simulink model "DEP_PROJECT"  (R2022b)
settings: Solver=VariableStepAuto  StartTime=0.0  StopTime=2
undefined symbols (not defined in the file): Ion, Lithium
libraries: spsMosfetLib x6, spsBatteryLib x1, spsPermanentMagnetSynchronousMachineLib x1, simulink x1, slpidlib x1, spspowerguiLib x1
settings Model: Creator=Deepak  LastModifiedBy=revat
settings SolverCC: AlgebraicLoopSolver=TrustRegion
settings DebuggingCC: UnconnectedInputMsg=warning  UnconnectedOutputMsg=warning  UnconnectedLineMsg=warning  SFMachineParentedDataDiag=warning
settings ModelReferenceCC: EnableRefExpFcnMdlSchedulingChecks=on
settings SFSimCC: CustomCodeUndefinedFunction=UseInterfaceOnly

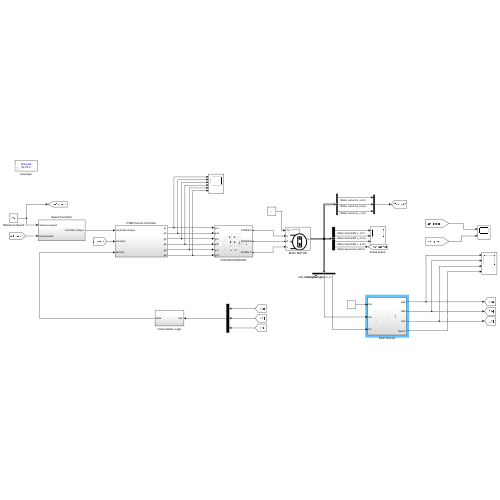
[thumbnail: Simulink's stored preview of the top-level diagram]
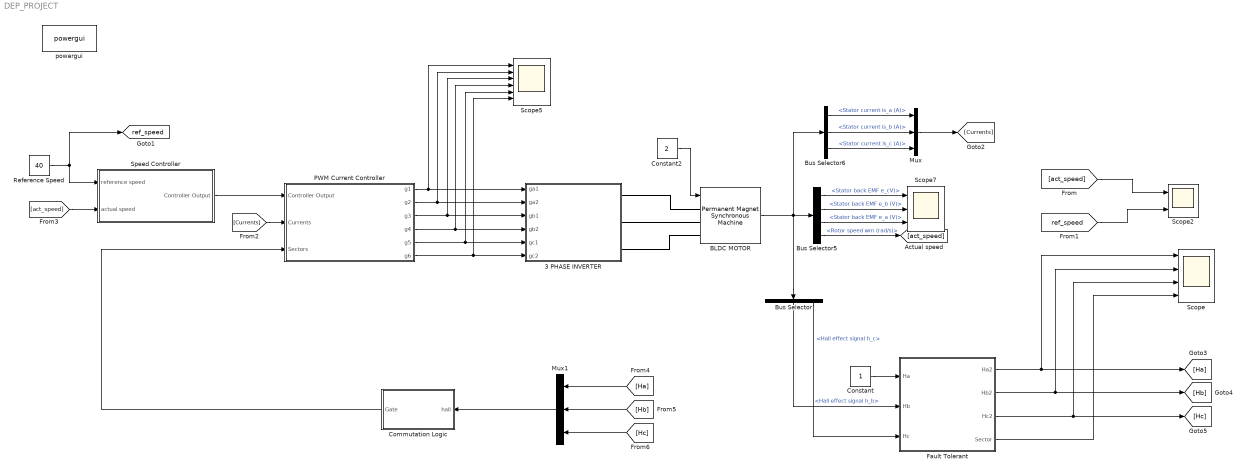
== system DEP_PROJECT ==
  3 PHASE INVERTER : Subsystem
  BLDC MOTOR : spsPermanentMagnetSynchronousMachineLib/Permanent Magnet Synchronous Machine  NbPhases=3  FluxDistribution=Trapezoidal  RotorType=Round  MechanicalLoad=Torque Tm  PresetModel=No  ShowDetailedParameters=on  MeasurementBus=off  Resistance=0.7  Inductance=2.7e-3  dqInductances=[8.5e-3,8.5e-3]  La=0.000395  MachineConstant=Flux linkage established by magnets (V.s)  Flux=0.1194  VoltageCst=100.0283  TorqueCst=0.9552  Flat=120  Mechanical=[0.0027 0.0004924 4 0]  PolePairs=4  InitialConditions=[0,0, 0,0]  InitialConditions5ph=[0 0 0 0 0 0]  RefAngle=90 degrees behind phase A axis (modified Park)  IterativeDiscreteModel=Trapezoidal non iterative  TsBlock=-1  TsPowergui=0
  Bus Selector : BusSelector  OutputSignals=Hall effect signal h_a,Hall effect signal h_b,Hall effect signal h_c
  Bus Selector5 : BusSelector  OutputSignals=Stator back EMF e_cV),Stator back EMF e_b (V),Stator back EMF e_a (V),Rotor speed wm (rad/s)
  Bus Selector6 : BusSelector  OutputSignals=Stator current is_a (A),Stator current is_b (A),Stator current is_c (A)
  Commutation Logic : Subsystem
  Constant : Constant
  Constant2 : Constant  Value=2
  Fault Tolerant : Subsystem
  Mux : Mux  Inputs=3
  Mux1 : Mux  Inputs=3
  PWM Current Controller : Subsystem
  Reference Speed : Constant  Value=40
  Scope : Scope  NumInputPorts=4
  Scope2 : Scope  NumInputPorts=2
  Scope5 : Scope  NumInputPorts=6
  Scope7 : Scope  NumInputPorts=3
  Speed Controller : Subsystem
  powergui : spspowerguiLib/powergui  Priority=1  SimulationMode=Discrete  SampleTime=50e-6  frequency=60  Iterations=50  frequencyindice=0  Pbase=100e6  ErrMax=1e-4  UnitsV=kV  UnitsW=MW  buscounter=0  FunctionMessages=off  echomessages=off  EnableUseOfTLC=off  CurrentSourceSwitches=off  DisableSnubberDevices=off  DisableRonSwitches=off  DisableVfSwitches=off  DisplayEquations=off  AutomaticDiscreteSolvers=off  SolverType=Tustin/Backward Euler (TBE)  Interpol=off  ExternalGateDelay=off  methode=off  Ts=100  x0status=blocks  SPID=on  SwTol=0  HookPort=off  NonlinearTolerance=0  nMaxIteration=15  ContinueOnMaxIteration=off  RestoreLinks=warning  ResistiveCurrentMeasurement=off  Frange=[0:2:500]  Ylog=off  Xlog=on  ShowGrid=off  save=off  variable=ZData  structure=0  ZoomFFT=off  StartTime=0.0  cycles=1  DisplayStyle=1  fundamental=60  FreqAxis=off  MaxFrequency=1000  frequencyindicesteady=1  RmsSteady=1  display=off
  tag scope: ref_speed=global
  wires:
  Constant2/1 -> BLDC MOTOR/1
  PWM Current Controller/3(g3) -> Scope5/3, 3 PHASE INVERTER/3(gb1)
  PWM Current Controller/2(g2) -> 3 PHASE INVERTER/2(ga2), Scope5/2
  Commutation Logic/1(Gate) -> PWM Current Controller/3(Sectors)
  Bus Selector6/3 -> Mux/3  "<Stator current is_c (A)>"
  Bus Selector6/2 -> Mux/2  "<Stator current is_b (A)>"
  Reference Speed/1 -> Speed Controller/1(reference speed), [ref_speed]
  Speed Controller/1("Controller Output ") -> PWM Current Controller/1("Controller Output ")
  Bus Selector5/3 -> Scope7/3  "<Stator back EMF e_a (V)>"
  PWM Current Controller/5(g5) -> Scope5/5, 3 PHASE INVERTER/5(gc1)
  Bus Selector5/2 -> Scope7/2  "<Stator back EMF e_b (V)>"
  Bus Selector6/1 -> Mux/1  "<Stator current is_a (A)>"
  PWM Current Controller/6(g6) -> 3 PHASE INVERTER/6(gc2), Scope5/6
  PWM Current Controller/4(g4) -> Scope5/4, 3 PHASE INVERTER/4(gb2)
  Bus Selector5/4 -> [act_speed]  "<Rotor speed wm (rad/s)>"
  BLDC MOTOR/1 -> Bus Selector5/1, Bus Selector/1, Bus Selector6/1
  PWM Current Controller/1(g1) -> 3 PHASE INVERTER/1(ga1), Scope5/1
  Bus Selector5/1 -> Scope7/1  "<Stator back EMF e_cV)>"
  Mux1/1 -> Commutation Logic/1("hall ")
  [act_speed] -> Scope2/1
  [Currents] -> PWM Current Controller/2(Currents)
  Mux/1 -> [Currents]
  [act_speed] -> Speed Controller/2(actual speed)
  Fault Tolerant/1(Ha2) -> Scope/1, [Ha]
  Fault Tolerant/2(Hb2) -> [Hb], Scope/2
  Fault Tolerant/3(Hc2) -> [Hc], Scope/3
  Fault Tolerant/4(Sector) -> Scope/4
  Bus Selector/3 -> Fault Tolerant/3(Hc)  "<Hall effect signal h_c>"
  [Ha] -> Mux1/1
  [Hb] -> Mux1/2
  [Hc] -> Mux1/3
  [ref_speed] -> Scope2/2
  Bus Selector/2 -> Fault Tolerant/2(Hb)  "<Hall effect signal h_b>"
  Constant/1 -> Fault Tolerant/1(Ha)
  connections:
  3 PHASE INVERTER/RConn3 -- BLDC MOTOR/LConn3
  3 PHASE INVERTER/RConn1 -- BLDC MOTOR/LConn1
  3 PHASE INVERTER/RConn2 -- BLDC MOTOR/LConn2

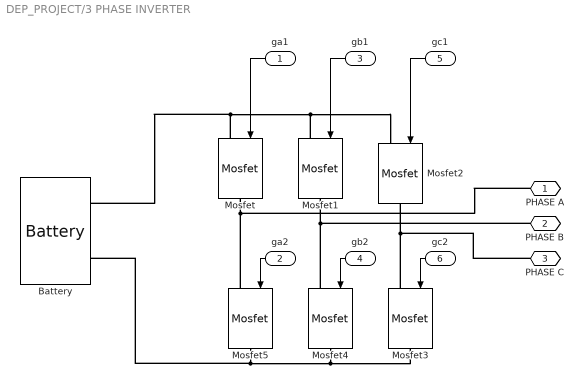
== system DEP_PROJECT/3 PHASE INVERTER ==
  ga1 : Inport
  ga2 : Inport  Port=2
  gb1 : Inport  Port=3
  gb2 : Inport  Port=4
  gc1 : Inport  Port=5
  gc2 : Inport  Port=6
  Battery : spsBatteryLib/Battery  BatType=Lithium-Ion  ShowTempParam=off  ThermalPreset=no  ShowAgeParam=off  NomV=48  NomQ=80  SOC=60  Batt_Tr=30  PresetModel=off  MaxQ=84  MinV=36  FullV=56.818272  Dis_rate=27.82608  R=0.006  Normal_OP=57.87524  expZone=[54.89208 3.144344]  current=[1.5 3]  Units=Ampere-hour  Tci=20  NomT=20  T2=-30  MaxQ2=4.8  FullV2=7.1  Normal_OP2=5.655  expZone2="[6.58           1]"  Rca=0.6  ti=2000  Dp=0  Neq0=0  Tsim=1e6  Ta1=25  Qeol=5.4*0.9  Reol=0.013333*1.2  Char_age=[2.3478, 3]  Dis_age=[2.3478, 10]  N1=1500  N2=10500  N3=1000  N4=1400  Ta2=45  N5=950
  Mosfet{,1..5} (6 alike) : spsMosfetLib/Mosfet  Ron=0.1  Lon=0  Rd=0.01  Vfd=0  IC=0  Rs=1e5  Cs=inf  Measurements=off
  PHASE A : PMIOPort  Side=Right
  PHASE B : PMIOPort  Port=2  Side=Right
  PHASE C : PMIOPort  Port=3  Side=Right
  wires:
  ga1/1 -> Mosfet/1
  ga2/1 -> Mosfet5/1
  gb1/1 -> Mosfet1/1
  gb2/1 -> Mosfet4/1
  gc1/1 -> Mosfet2/1
  gc2/1 -> Mosfet3/1
  connections:
  Mosfet5/LConn1 -- PHASE A/RConn1 -- Mosfet/RConn1
  PHASE B/RConn1 -- Mosfet4/LConn1 -- Mosfet1/RConn1
  Mosfet3/LConn1 -- PHASE C/RConn1 -- Mosfet2/RConn1
  Mosfet5/RConn1 -- Battery/LConn2 -- Mosfet4/RConn1 -- Mosfet3/RConn1
  Mosfet/LConn1 -- Battery/LConn1 -- Mosfet1/LConn1 -- Mosfet2/LConn1

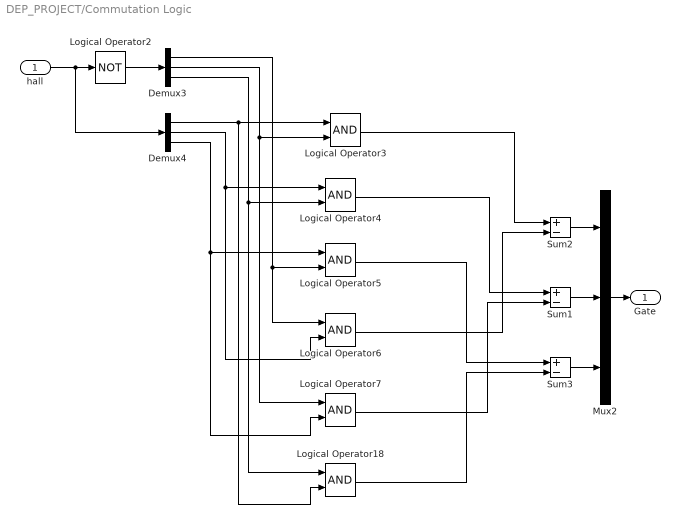
== system DEP_PROJECT/Commutation Logic ==
  "hall " : Inport
  Demux3 : Demux  Outputs=3
  Demux4 : Demux  Outputs=3
  Logical Operator{3..7,18} (6 alike) : Logic  AllPortsSameDT=off  OutDataTypeStr=boolean
  Logical Operator2 : Logic  Operator=NOT  AllPortsSameDT=off  OutDataTypeStr=boolean
  Mux2 : Mux  Inputs=3
  Sum1 : Sum  Inputs=+-  OutDataTypeStr=double
  Sum2 : Sum  Inputs=+-  OutDataTypeStr=double
  Sum3 : Sum  Inputs=+-  OutDataTypeStr=double
  Gate : Outport  VectorParamsAs1DForOutWhenUnconnected=off
  wires:
  Demux3/3 -> Logical Operator18/1, Logical Operator4/2
  Logical Operator6/1 -> Sum2/2
  Mux2/1 -> Gate/1
  Logical Operator7/1 -> Sum1/2
  Logical Operator4/1 -> Sum1/1
  Demux4/1 -> Logical Operator18/2, Logical Operator3/1
  Sum2/1 -> Mux2/1
  Demux4/3 -> Logical Operator5/1, Logical Operator7/2
  Demux4/2 -> Logical Operator4/1, Logical Operator6/2
  Logical Operator5/1 -> Sum3/1
  Logical Operator3/1 -> Sum2/1
  Sum1/1 -> Mux2/2
  Demux3/1 -> Logical Operator5/2, Logical Operator6/1
  Logical Operator2/1 -> Demux3/1
  Logical Operator18/1 -> Sum3/2
  Demux3/2 -> Logical Operator7/1, Logical Operator3/2
  "hall "/1 -> Logical Operator2/1, Demux4/1
  Sum3/1 -> Mux2/3

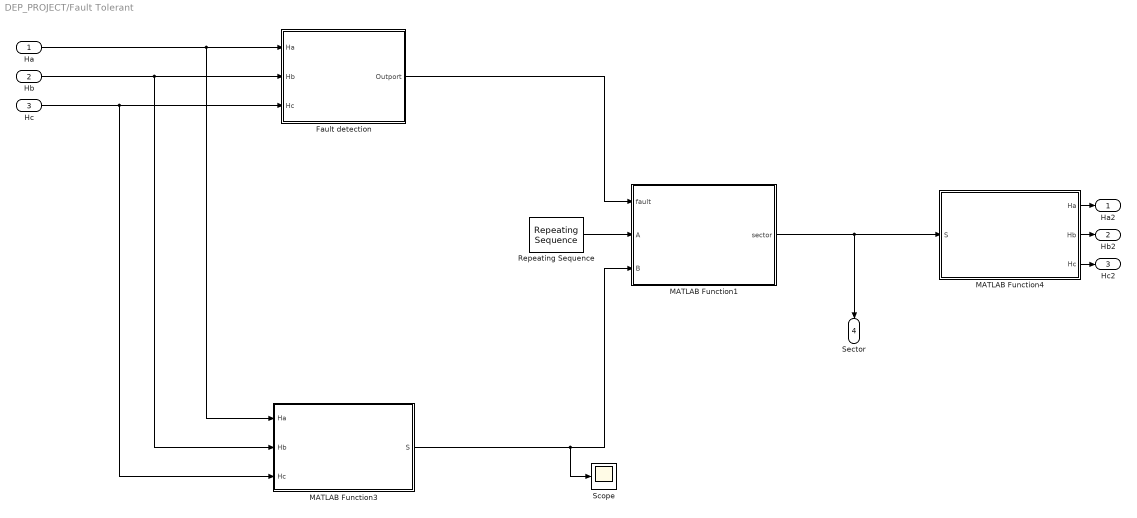
== system DEP_PROJECT/Fault Tolerant ==
  Ha : Inport
  Hb : Inport  Port=2
  Hc : Inport  Port=3
  Fault detection : Subsystem
  MATLAB Function1 : MATLAB Function  TreatAsAtomicUnit=on
  MATLAB Function3 : MATLAB Function  TreatAsAtomicUnit=on
  MATLAB Function4 : MATLAB Function  TreatAsAtomicUnit=on
  Repeating Sequence : simulink/Sources/Repeating Sequence  rep_seq_t=[0 8.799 8.8 17.59999 17.6 26.39999 26.4 35.1999 35.2 43.9999 44 52.79999 52.8]*(6.616/8.8)*1e-03  rep_seq_y=[1 1 2 2 3 3 4 4 5 5 6 6 1]
  Scope : Scope
  Ha2 : Outport
  Hb2 : Outport  Port=2
  Hc2 : Outport  Port=3
  Sector : Outport  Port=4
  wires:
  Hb/1 -> MATLAB Function3/2(Hb), Fault detection/2(Hb)
  Fault detection/1(Outport) -> MATLAB Function1/1(fault)
  MATLAB Function3/1(S) -> Scope/1, MATLAB Function1/3(B)
  MATLAB Function4/3(Hc) -> Hc2/1
  Hc/1 -> MATLAB Function3/3(Hc), Fault detection/3(Hc)
  MATLAB Function4/1(Ha) -> Ha2/1
  MATLAB Function1/1(sector) -> Sector/1, MATLAB Function4/1(S)
  Ha/1 -> MATLAB Function3/1(Ha), Fault detection/1(Ha)
  MATLAB Function4/2(Hb) -> Hb2/1
  Repeating Sequence/1 -> MATLAB Function1/2(A)

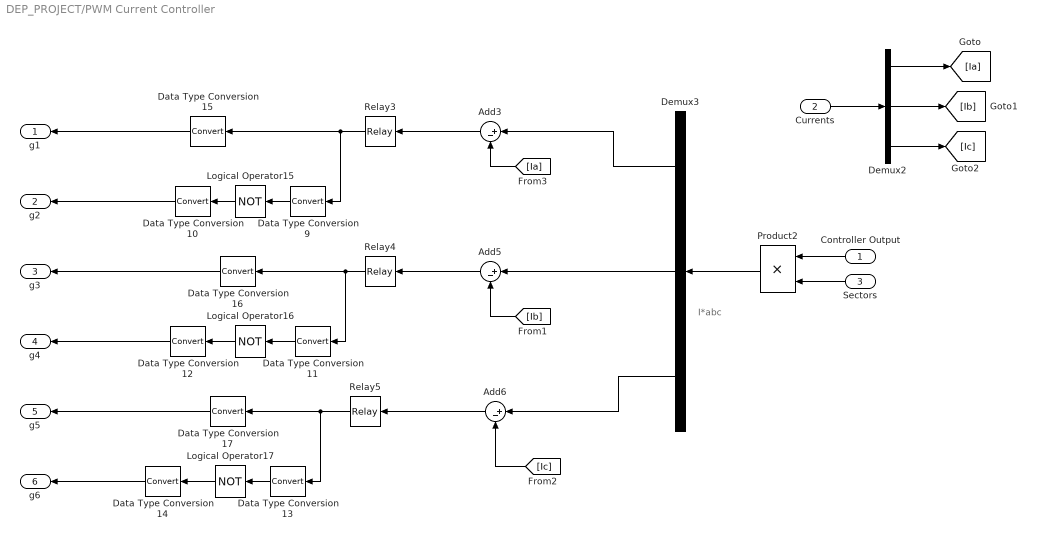
== system DEP_PROJECT/PWM Current Controller ==
  note: I*abc
  "Controller Output " : Inport
  Currents : Inport  Port=2
  Sectors : Inport  Port=3
  Add3 : Sum  Inputs=|+-
  Add5 : Sum  Inputs=|+-
  Add6 : Sum  Inputs=|+-
  Data Type Conversion{9..17} (9 alike) : DataTypeConversion
  Demux2 : Demux  Outputs=3
  Demux3 : Demux  Outputs=3
      settings: DisplayOption=none
  Logical Operator15 : Logic  Operator=NOT  AllPortsSameDT=off  OutDataTypeStr=boolean
  Logical Operator16 : Logic  Operator=NOT  AllPortsSameDT=off  OutDataTypeStr=boolean
  Logical Operator17 : Logic  Operator=NOT  AllPortsSameDT=off  OutDataTypeStr=boolean
  Product2 : Product  SaturateOnIntegerOverflow=on  OutDataTypeStr=Inherit: Same as first input
  Relay3 : Relay  OnSwitchValue=0.1  OffSwitchValue=-0.1
  Relay4 : Relay  OnSwitchValue=0.1  OffSwitchValue=-0.1
  Relay5 : Relay  OnSwitchValue=0.1  OffSwitchValue=-0.1
  g1 : Outport  VectorParamsAs1DForOutWhenUnconnected=off
  g2 : Outport  Port=2  VectorParamsAs1DForOutWhenUnconnected=off
  g3 : Outport  Port=3  VectorParamsAs1DForOutWhenUnconnected=off
  g4 : Outport  Port=4  VectorParamsAs1DForOutWhenUnconnected=off
  g5 : Outport  Port=5  VectorParamsAs1DForOutWhenUnconnected=off
  g6 : Outport  Port=6  VectorParamsAs1DForOutWhenUnconnected=off
  wires:
  Currents/1 -> Demux2/1
  Demux2/1 -> [Ia]
  Demux2/2 -> [Ib]
  Demux2/3 -> [Ic]
  "Controller Output "/1 -> Product2/1
  Sectors/1 -> Product2/2
  Add6/1 -> Relay5/1
  Add5/1 -> Relay4/1
  Demux3/1 -> Add3/1
  Data Type Conversion16/1 -> g3/1
  Data Type Conversion13/1 -> Logical Operator17/1
  Add3/1 -> Relay3/1
  Product2/1 -> Demux3/1
  Relay3/1 -> Data Type Conversion15/1, Data Type Conversion9/1
  Data Type Conversion15/1 -> g1/1
  Relay4/1 -> Data Type Conversion16/1, Data Type Conversion11/1
  Data Type Conversion17/1 -> g5/1
  Data Type Conversion12/1 -> g4/1
  Data Type Conversion10/1 -> g2/1
  Data Type Conversion11/1 -> Logical Operator16/1
  [Ic] -> Add6/2
  Logical Operator17/1 -> Data Type Conversion14/1
  Data Type Conversion14/1 -> g6/1
  Demux3/2 -> Add5/1
  Relay5/1 -> Data Type Conversion17/1, Data Type Conversion13/1
  Logical Operator15/1 -> Data Type Conversion10/1
  Logical Operator16/1 -> Data Type Conversion12/1
  [Ia] -> Add3/2
  Demux3/3 -> Add6/1
  Data Type Conversion9/1 -> Logical Operator15/1
  [Ib] -> Add5/2

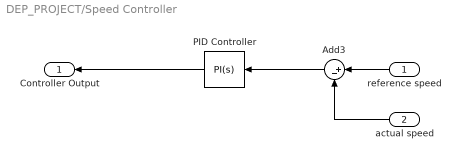
== system DEP_PROJECT/Speed Controller ==
  reference speed : Inport
  actual speed : Inport  Port=2
  Add3 : Sum  Inputs=|+-
  PID Controller : slpidlib/PID Controller  Controller=PI  Form=Parallel  TimeDomain=Continuous-time  UseExternalTs=off  SampleTime=-1  IntegratorMethod=Forward Euler  FilterMethod=Forward Euler  ControllerParametersSource=internal  P=5  I=4.9  UseKiTs=off  D=0  N=100  UseFilter=on  TunerSelectOption=Transfer Function Based (PID Tuner App)  InitialConditionSource=internal  InitialConditionForIntegrator=0  InitialConditionForFilter=0  DifferentiatorICPrevScaledInput=0  ExternalReset=none  TrackingMode=off  Kt=1  LimitOutput=off  SatLimitsSource=internal  UpperSaturationLimit=10  LowerSaturationLimit=0  LinearizeAsGain=on  AntiWindupMode=none  Kb=1  LimitIntegrator=off  UpperIntegratorSaturationLimit=inf  LowerIntegratorSaturationLimit=-inf  POutMin=[]  POutMax=[]  IOutMin=[]  IOutMax=[]  DOutMin=[]  DOutMax=[]  NOutMin=[]  NOutMax=[]  SumOutMin=[]  SumOutMax=[]  SaturationOutMin=[]  SaturationOutMax=[]  PParamMin=[]  PParamMax=[]  IParamMin=[]  IParamMax=[]  DParamMin=[]  DParamMax=[]  NParamMin=[]  NParamMax=[]  KbParamMin=[]  KbParamMax=[]  KtParamMin=[]  KtParamMax=[]  KbOutMin=[]  KbOutMax=[]  KtOutMin=[]  KtOutMax=[]  IntegratorOutMin=[]  IntegratorOutMax=[]  FilterOutMin=[]  FilterOutMax=[]  SumI1OutMin=[]  SumI1OutMax=[]  SumI2OutMin=[]  SumI2OutMax=[]  SumI3OutMin=[]  SumI3OutMax=[]  SumI4OutMin=[]  SumI4OutMax=[]  SumDOutMin=[]  SumDOutMax=[]  DifferentiatorOutMin=[]  DifferentiatorOutMax=[]  FilterDiffOutCoefMin=[]  FilterDiffOutCoefMax=[]  ReciprocalOutMin=[]  ReciprocalOutMax=[]  SumDenOutMin=[]  SumDenOutMax=[]  SumNumOutMin=[]  SumNumOutMax=[]  DivideOutMin=[]  DivideOutMax=[]  UdiffTsProdOutMin=[]  UdiffTsProdOutMax=[]  NTsProdOutMin=[]  NTsProdOutMax=[]  UintegralTsProdOutMin=[]  UintegralTsProdOutMax=[]  UngainTsProdOutMin=[]  UngainTsProdOutMax=[]  ClampingZeroOutDataTypeStr=Inherit: Inherit via back propagation  ClampingZeroOutMin=[]  ClampingZeroOutMax=[]  FilterDenConstantOutDataTypeStr=Inherit: Inherit via back propagation  FilterDenConstantOutMin=[]  FilterDenConstantOutMax=[]  PCopyOutDataTypeStr=Inherit: Inherit via back propagation  PCopyOutMin=[]  PCopyOutMax=[]  NCopyOutDataTypeStr=Inherit: Inherit via back propagation  NCopyOutMin=[]  NCopyOutMax=[]  IntegratorContinuousStateAttributes=''  IntegratorStateMustResolveToSignalObject=off  IntegratorRTWStateStorageClass=Auto  FilterContinuousStateAttributes=''  FilterStateMustResolveToSignalObject=off  FilterRTWStateStorageClass=Auto  ParallelPVariant=InternalParameters  IdealPVariant=Disabled  IVariant=InternalParameters  DVariant=Disabled  IntegratorVariant=Continuous  SatVariant=Disabled  AWVariant=Passthrough  PCopyVariant=Disabled  TRVariant=Disabled  FdbkBlocksVariant=Forward  IdealPFdbkVariant=Disabled  SatFdbkVariant=Disabled  DerivativeFilterVariant=Disabled  NVariant=Disabled  NCopyVariant=Disabled_SignalSpec  FilterICVariant=Disabled  IntegratorICVariant=InternalICs  ExternalResetVariant=Disabled  TRSumVariant=Passthrough  SumFdbkVariant=Disabled  SumVariant=Sum_PI  TsampFilterVariant=InternalTs  TsampNgainVariant=Passthrough  TsampIntegralVariant=Passthrough  ExternalSaturationOutDataTypeStr=Inherit: Same as second input
  "Controller Output " : Outport  VectorParamsAs1DForOutWhenUnconnected=off
  wires:
  Add3/1 -> PID Controller/1
  actual speed/1 -> Add3/2
  PID Controller/1 -> "Controller Output "/1
  reference speed/1 -> Add3/1

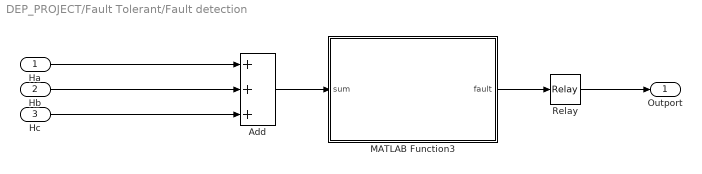
== system DEP_PROJECT/Fault Tolerant/Fault detection ==
  Ha : Inport
  Hb : Inport  Port=2
  Hc : Inport  Port=3
  Add : Sum  Inputs=+++
  MATLAB Function3 : MATLAB Function  TreatAsAtomicUnit=on
  Relay : Relay  OnSwitchValue=1  OffSwitchValue=-1
  Outport : Outport
  wires:
  MATLAB Function3/1(fault) -> Relay/1
  Add/1 -> MATLAB Function3/1(sum)
  Ha/1 -> Add/1
  Hc/1 -> Add/3
  Hb/1 -> Add/2
  Relay/1 -> Outport/1

== matlab function DEP_PROJECT/Fault Tolerant/MATLAB Function1 ==
  data: sector output; fault input; A input; B input
function sector= final(fault,A,B)

if fault ==1
    sector=A;

else 
    sector = B;

end

== matlab function DEP_PROJECT/Fault Tolerant/MATLAB Function3 ==
  data: S output; Ha input; Hb input; Hc input
function S = get_motor_state(Ha,Hb,Hc)
S=0;
if (Ha==0)&&(Hb==0)&&(Hc==0)
    S=0;
end
if (Ha==1)&&(Hb==1)&&(Hc==0)
    S=1;
end
if (Ha==0)&&(Hb==1)&&(Hc==0)
     S=2;
end
if (Ha==0)&&(Hb==1)&&(Hc==1)
    S=3;
end
if (Ha==0)&&(Hb==0)&&(Hc==1)
     S=4;
end
if (Ha==1)&&(Hb==0)&&(Hc==1)
     S=5;
end
if (Ha==1)&&(Hb==0)&&(Hc==0)
     S=6;
end
if (Ha==1)&&(Hb==1)&&(Hc==1)
     S=7;
end
end

== matlab function DEP_PROJECT/Fault Tolerant/Fault detection/MATLAB Function3 ==
  data: fault output; sum input
function fault = fault_det(sum)
if sum==0 || sum==3
   fault=1;
else 
    fault=0;
end
end

== matlab function DEP_PROJECT/Fault Tolerant/MATLAB Function4 ==
  data: Ha output; S input; Hb output; Hc output
function [Ha,Hb,Hc] = hall(S)
Ha=0;
Hb=0;
Hc=0;
if S==0
    Ha=0; Hb=0; Hc=0;
    
end
if S==1
    Ha=1; Hb=1; Hc=0;
    
end
if S==2
    Ha=0; Hb=1; Hc=0;
    
end
if S==3
    Ha=0; Hb=1; Hc=1;
    
end
if S==4
    Ha=0; Hb=0; Hc=1;
    
end
if S==5
    Ha=1; Hb=0; Hc=1;
    
end
if S==6
    Ha=1; Hb=0; Hc=0;
    
end
if S==7
    Ha=1; Hb=1; Hc=1;
    
end
end
